simulink subsystem "Plant"  (R2024b)
settings: Solver=VariableStepAuto  StartTime=0.0  StopTime=10.0  RelTol=1e-3
model mask{initial_data=launch_initial, maneuver_time=0, mu=Earth_planet.mu}
  mask prompts: initial_data "Initial Data"; maneuver_time "Gravity Switch Time"; mu "Gravitational Parameter"
values from neighbouring files (symbols this model uses):
  mu = G*M    (= 398704760000000)    [Earth_setup.m]    (also in Mars_capture_setup.m = 4.2840406e+13; Mars_setup.m = 4.2840406e+13)
libraries: vrlib x1
settings Model: Creator=cpero  LastModifiedBy=cpero

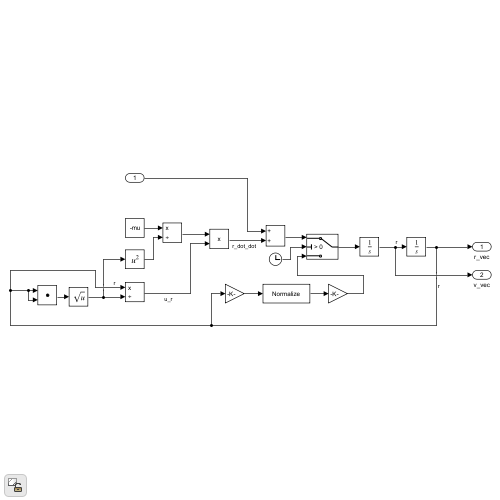
[thumbnail: Simulink's stored preview of the top-level diagram]
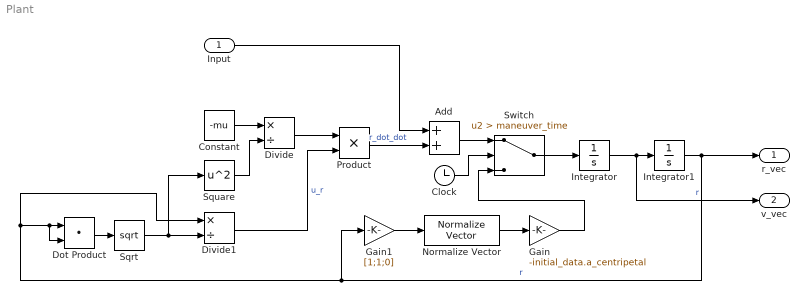
== system Plant ==
  Input : Inport
  Add : Sum
  Clock : Clock
  Constant : Constant  Value=-mu
  Divide : Product  Inputs=*/
  Divide1 : Product  Inputs=*/
  Dot Product : DotProduct  OutDataTypeStr=Inherit: Inherit via internal rule
  Gain : Gain  Gain=-initial_data.a_centripetal
  Gain1 : Gain  Gain=[1;1;0]
  Integrator : Integrator  InitialCondition=initial_data.v_initial
  Integrator1 : Integrator  InitialCondition=initial_data.r_initial
  Normalize Vector : vrlib/Utilities/Normalize Vector  maxzero=0
  Product : Product
  Sqrt : Sqrt
  Square : Math  Operator=square
  Switch : Switch  Criteria=u2 > Threshold  Threshold=maneuver_time  ZeroCross=off  SaturateOnIntegerOverflow=off  InputSameDT=off
  r_vec : Outport
  v_vec : Outport  Port=2
  wires:
  Integrator1/1 -> r_vec/1, Divide1/1, Dot Product/1, Dot Product/2, Gain1/1  "r"
  Divide1/1 -> Product/2  "u_r"
  Sqrt/1 -> Divide1/2, Square/1
  Divide/1 -> Product/1
  Square/1 -> Divide/2
  Dot Product/1 -> Sqrt/1
  Constant/1 -> Divide/1
  Product/1 -> Add/2  "r_dot_dot"
  Switch/1 -> Integrator/1
  Add/1 -> Switch/1
  Clock/1 -> Switch/2
  Normalize Vector/1 -> Gain/1
  Gain/1 -> Switch/3
  Gain1/1 -> Normalize Vector/1
  Integrator/1 -> Integrator1/1, v_vec/1  "r"
  Input/1 -> Add/1
